simulink model "pt8612pll_4"  (Simulink 5.0)
settings: Solver=ode45  StartTime=0.0  StopTime=50  RelTol=1e-8  AbsTol=1e-11
values from neighbouring files (symbols this model uses):
  C = 680e-9    (= 6.8e-07)    [PT8612PLLinit.m]    (also in PT8612PLLinit_2.m; PT8612PLLinit_3.m; PT8612PLLinit_4.m; colorimetry_rom.m = [[CrCgCb(1) 0 0];[0 CrCgCb(2) 0];[0 0 CrCgCb(3)]])
  fvcxo = 148.5e6/1.001    (= 148351648.352)    [PT8612PLLinit.m]    (also in PT8612PLLinit_2.m; PT8612PLLinit_3.m; PT8612PLLinit_4.m)
  Gp = 1/4    (= 0.25)    [PT8612PLLinit.m]    (also in PT8612PLLinit_2.m = 0.025; PT8612PLLinit_4.m = 256)
  Kvcxo = 90e-6    (= 9e-05)    [PT8612PLLinit.m]    (also in PT8612PLLinit_2.m; PT8612PLLinit_3.m; PT8612PLLinit_4.m)
  Nbdac = Nbl    (= 20)    [PT8612PLLinit_4.m]
  Nbl = 20    [PT8612PLLinit_4.m]
  Nblint = 24    [PT8612PLLinit_4.m]
  Nfodiv = 500*4    (= 2000)    [PT8612PLLinit_2.m]    (also in PT8612PLLinit_3.m; PT8612PLLinit_4.m = 500000)
  R = 100e3    (= 100000)    [PT8612PLLinit.m]    (also in PT8612PLLinit_2.m = 220000; PT8612PLLinit_3.m = 82000; PT8612PLLinit_4.m = 200000; combi_signal.m = [R;ones(red_heigth,spl)])
  Tsi = Tsloop    (= 0.00337037037037)    [PT8612PLLinit_4.m]
  Tsloop = 1/fvcxo*Nfodiv    (= 0.00337037037037)    [PT8612PLLinit_4.m]
  Vcc = 3.3    [PT8612PLLinit_2.m]    (also in PT8612PLLinit_3.m; PT8612PLLinit_4.m)
libraries: simulink x3
settings Model: LastModifiedBy=thh

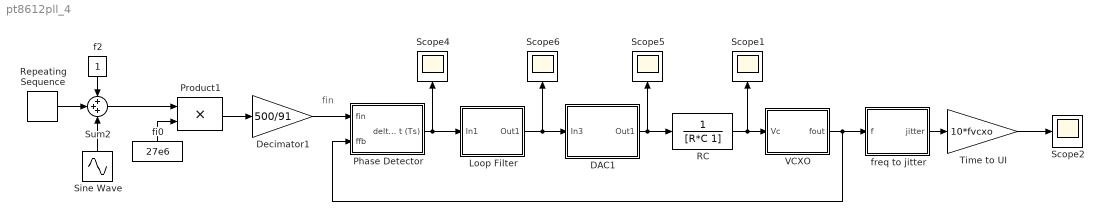
== system pt8612pll_4 ==
  note: fin
  DAC1 : Subsystem
  Decimator1 : Gain  Gain=500/91  SaturateOnIntegerOverflow=on
  Loop Filter : Subsystem
  Phase Detector : Subsystem
  Product1 : Product  SaturateOnIntegerOverflow=on
  RC : TransferFcn  Denominator=[R*C 1]
  Repeating Sequence : simulink/Sources/Repeating Sequence  rep_seq_t=[0 50 50 100]  rep_seq_y=[-1 -1 1 1]*0e-6
  Scope{1..2,4..6} (5 alike) : Scope
      Scope1 settings: Orientation=up  TimeRange=10  YMin=1.24775  YMax=1.2525
      Scope2 settings: TimeRange=13.94281180037974  YMin=4.875047510948617  YMax=5.128263723388365  SaveName=ScopeData3
      Scope4 settings: Orientation=up  TimeRange=10  YMin=-0.5  YMax=0.5
      Scope5 settings: Orientation=up  TimeRange=10  YMin=1.175  YMax=1.55  SaveName=ScopeData5
      Scope6 settings: Orientation=up  TimeRange=10  YMax=25  SaveName=ScopeData6
  Sine Wave : Sin  Orientation=up  Amplitude=0e-6  SampleTime=0
  Sum2 : Sum  Inputs=+++  SaturateOnIntegerOverflow=on
  Time to UI : Gain  Gain=10*fvcxo  SaturateOnIntegerOverflow=on
  VCXO : Subsystem
  f2 : Constant  Orientation=down
  fi0 : Constant  Orientation=up  Value=27e6
  freq to jitter : Subsystem
  wires:
  Phase Detector/1(delta t (Ts)) -> Scope4/1, Loop Filter/1(In1)
  VCXO/1(fout) -> freq to jitter/1(f), Phase Detector/2(ffb)
  Product1/1 -> Decimator1/1
  f2/1 -> Sum2/1
  Sum2/1 -> Product1/1
  Repeating Sequence/1 -> Sum2/2
  Loop Filter/1(Out1) -> DAC1/1(In3), Scope6/1
  freq to jitter/1(jitter) -> Time to UI/1
  fi0/1 -> Product1/2
  Time to UI/1 -> Scope2/1
  Decimator1/1 -> Phase Detector/1(fin)
  DAC1/1(Out1) -> Scope5/1, RC/1
  RC/1 -> Scope1/1, VCXO/1(Vc)
  Sine Wave/1 -> Sum2/3

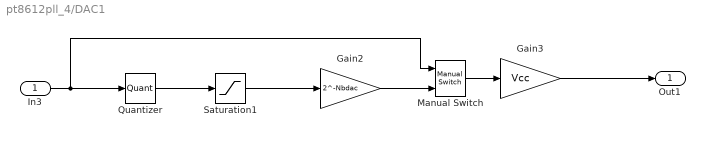
== system pt8612pll_4/DAC1 ==
  In3 : Inport
  Gain2 : Gain  Gain=2^-Nbdac  SaturateOnIntegerOverflow=on
  Gain3 : Gain  Gain=Vcc  SaturateOnIntegerOverflow=on
  Manual Switch : simulink/Signal Routing/Manual Switch  sw=0  action=0
  Quantizer : Quantizer  QuantizationInterval=1
  Saturation1 : Saturate  UpperLimit=2^Nbdac-1  LowerLimit=0
  Out1 : Outport
  wires:
  In3/1 -> Manual Switch/1, Quantizer/1
  Quantizer/1 -> Saturation1/1
  Gain2/1 -> Manual Switch/2
  Manual Switch/1 -> Gain3/1
  Gain3/1 -> Out1/1
  Saturation1/1 -> Gain2/1

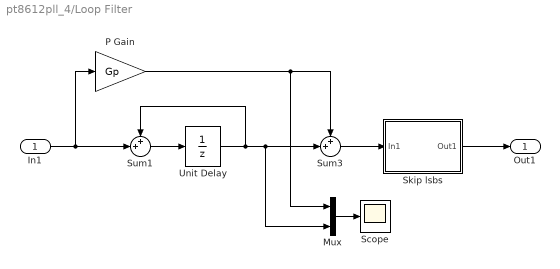
== system pt8612pll_4/Loop Filter ==
  In1 : Inport
  Mux : Mux  Inputs=2
  P Gain : Gain  Gain=Gp  SaturateOnIntegerOverflow=on
  Scope : Scope
      settings: YMin=-2.5e+006  YMax=5e+006  SaveName=ScopeData2
  Skip lsbs : Subsystem
  Sum1 : Sum  Inputs=++|  SaturateOnIntegerOverflow=on
  Sum3 : Sum  Inputs=++|  SaturateOnIntegerOverflow=on
  Unit Delay : UnitDelay  SampleTime=Tsi
  Out1 : Outport
  wires:
  P Gain/1 -> Sum3/1, Mux/1
  Sum3/1 -> Skip lsbs/1(In1)
  Mux/1 -> Scope/1
  Unit Delay/1 -> Sum3/2, Mux/2, Sum1/1
  Sum1/1 -> Unit Delay/1
  In1/1 -> P Gain/1, Sum1/2
  Skip lsbs/1(Out1) -> Out1/1

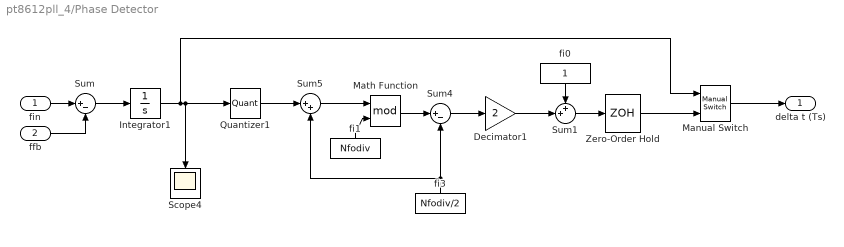
== system pt8612pll_4/Phase Detector ==
  fin : Inport
  ffb : Inport  Port=2
  Decimator1 : Gain  Gain=2  SaturateOnIntegerOverflow=on
  Integrator1 : Integrator
  Manual Switch : simulink/Signal Routing/Manual Switch  sw=0  action=0
  Math Function : Math  Operator=mod
  Quantizer1 : Quantizer  QuantizationInterval=1
  Scope4 : Scope
      settings: Orientation=down  TimeRange=10  YMin=-0.5  YMax=0.5  SaveName=ScopeData4
  Sum : Sum  Inputs=|+-  SaturateOnIntegerOverflow=on
  Sum1 : Sum  Inputs=++|  SaturateOnIntegerOverflow=on
  Sum4 : Sum  Inputs=|+-  SaturateOnIntegerOverflow=on
  Sum5 : Sum  Inputs=|++  SaturateOnIntegerOverflow=on
  Zero-Order Hold : ZeroOrderHold  SampleTime=Tsloop
  fi0 : Constant  Orientation=down
  fi1 : Constant  Orientation=up  Value=Nfodiv
  fi3 : Constant  Orientation=up  Value=Nfodiv/2
  delta t (Ts) : Outport
  wires:
  Sum/1 -> Integrator1/1
  fin/1 -> Sum/1
  ffb/1 -> Sum/2
  Integrator1/1 -> Manual Switch/1, Scope4/1, Quantizer1/1
  fi0/1 -> Sum1/1
  Sum1/1 -> Zero-Order Hold/1
  Zero-Order Hold/1 -> Manual Switch/2
  Manual Switch/1 -> delta t (Ts)/1
  Decimator1/1 -> Sum1/2
  fi1/1 -> Math Function/2
  Sum5/1 -> Math Function/1
  fi3/1 -> Sum4/2, Sum5/2
  Math Function/1 -> Sum4/1
  Sum4/1 -> Decimator1/1
  Quantizer1/1 -> Sum5/1

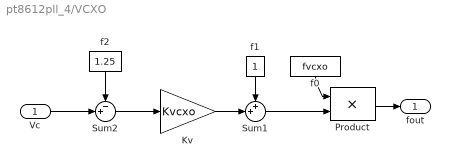
== system pt8612pll_4/VCXO ==
  Vc : Inport
  Kv : Gain  Gain=Kvcxo  SaturateOnIntegerOverflow=on
  Product : Product  SaturateOnIntegerOverflow=on
  Sum1 : Sum  Inputs=++|  SaturateOnIntegerOverflow=on
  Sum2 : Sum  Inputs=-+|  SaturateOnIntegerOverflow=on
  f0 : Constant  Orientation=down  Value=fvcxo
  f1 : Constant  Orientation=down
  f2 : Constant  Orientation=down  Value=1.25
  fout : Outport
  wires:
  f0/1 -> Product/1
  f1/1 -> Sum1/1
  Sum1/1 -> Product/2
  Kv/1 -> Sum1/2
  Product/1 -> fout/1
  Sum2/1 -> Kv/1
  Vc/1 -> Sum2/2
  f2/1 -> Sum2/1

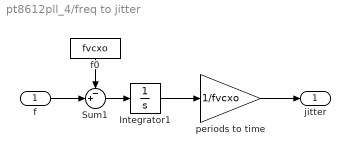
== system pt8612pll_4/freq to jitter ==
  f : Inport
  Integrator1 : Integrator
  Sum1 : Sum  Inputs=-+|  SaturateOnIntegerOverflow=on
  f0 : Constant  Orientation=down  Value=fvcxo
  periods to time : Gain  Gain=1/fvcxo  SaturateOnIntegerOverflow=on
  jitter : Outport
  wires:
  Integrator1/1 -> periods to time/1
  Sum1/1 -> Integrator1/1
  f0/1 -> Sum1/1
  f/1 -> Sum1/2
  periods to time/1 -> jitter/1

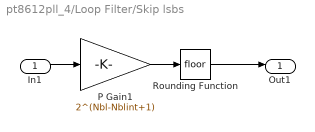
== system pt8612pll_4/Loop Filter/Skip lsbs ==
  In1 : Inport
  P Gain1 : Gain  Gain=2^(Nbl-Nblint+1)  SaturateOnIntegerOverflow=on
  Rounding Function : Rounding
  Out1 : Outport
  wires:
  P Gain1/1 -> Rounding Function/1
  In1/1 -> P Gain1/1
  Rounding Function/1 -> Out1/1
